simulink model "dec_fir_xblock"  (Simulink 7.4)
settings: Solver=ode45  StartTime=0.0  StopTime=10.0  RelTol=1e-3
libraries: xbsIndex_r4 x18, casper_library_misc x1
settings Model: Creator=chenhong  LastModifiedBy=chenhong

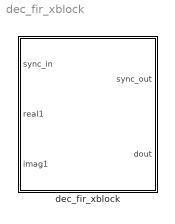
== system dec_fir_xblock ==
  dec_fir_xblock : Subsystem  mask{n_inputs=1, coeff=[0 0], n_bits=4, quantization=Truncate, add_latency=1, mult_latency=2, coeff_bit_width=25, coeff_bin_pt=24, adder_tree_hdl=on}
      mask prompts: n_inputs "Number of Parallel Streams"; coeff "Coefficients"; n_bits "Bit Width Out"; quantization "Quantization Behavior"; add_latency "Add Latency"; mult_latency "Mult Latency"; coeff_bit_width "Coefficient bit width"; coeff_bin_pt "Coefficient binary point"; adder_tree_hdl "Implement first stage of adder trees after multiplication as behavioural HDL"
      mask init:
      | config.source=str2func('dec_fir_init_xblock');
      | config.toplevel=gcb;
      | xBlock(config, ...
      |         {n_inputs,coeff,n_bits,quantization,add_latency,...
      |          mult_latency, coeff_bit_width,coeff_bin_pt,adder_tree_hdl})
      mask StyleString: edit,edit,edit,popup(Truncate|Round  (unbiased: +/- Inf)|Round  (unbiased: Even Values)),edit,edit,edit,edit,checkbox

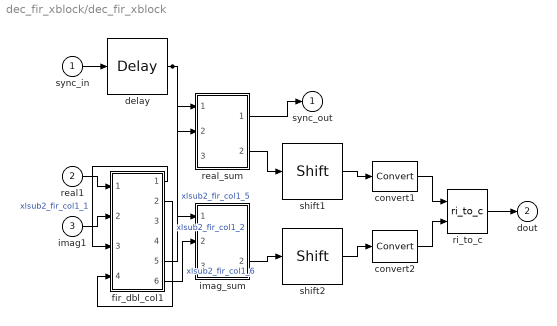
== system dec_fir_xblock/dec_fir_xblock ==
  sync_in : Inport
  real1 : Inport  Port=2
  imag1 : Inport  Port=3
  convert1 : xbsIndex_r4/Convert  arith_type="Signed  (2's comp)"  n_bits=4  bin_pt=3  quantization=Truncate  overflow=Wrap  latency=1  dbl_ovrd=off  pipeline=off  block_type=convert
      settings: block_version=11.4
  convert2 : xbsIndex_r4/Convert  arith_type="Signed  (2's comp)"  n_bits=4  bin_pt=3  quantization=Truncate  overflow=Wrap  latency=1  dbl_ovrd=off  pipeline=off  block_type=convert
      settings: block_version=11.4
  delay : xbsIndex_r4/Delay  en=off  latency=4  dbl_ovrd=off  reg_retiming=off  block_type=delay
      settings: block_version=11.4
  fir_dbl_col1 : Subsystem
  imag_sum : Subsystem
  real_sum : Subsystem
  ri_to_c : casper_library_misc/ri_to_c  SystemSampleTime=-1
  shift1 : xbsIndex_r4/Shift  shift_dir=Left  shift_bits=1  en=off  latency=0  precision=Full  arith_type="Signed  (2's comp)"  n_bits=16  bin_pt=14  quantization=Truncate  overflow=Wrap  dbl_ovrd=off  block_type=shift
  shift2 : xbsIndex_r4/Shift  shift_dir=Left  shift_bits=1  en=off  latency=0  precision=Full  arith_type="Signed  (2's comp)"  n_bits=16  bin_pt=14  quantization=Truncate  overflow=Wrap  dbl_ovrd=off  block_type=shift
  sync_out : Outport
  dout : Outport  Port=2
  wires:
  delay/1 -> real_sum/1(sync), imag_sum/1(sync)
  shift2/1 -> convert2/1
  imag_sum/2(dout) -> shift2/1
  shift1/1 -> convert1/1
  real_sum/2(dout) -> shift1/1
  ri_to_c/1 -> dout/1
  convert2/1 -> ri_to_c/2
  convert1/1 -> ri_to_c/1
  real_sum/1(sync_out) -> sync_out/1
  fir_dbl_col1/5(real_sum) -> real_sum/2(din_1)  "xlsub2_fir_col1_5"
  fir_dbl_col1/6(imag_sum) -> imag_sum/2(din_1)  "xlsub2_fir_col1_6"
  fir_dbl_col1/2(imag_out1) -> fir_dbl_col1/4(imag_back1)  "xlsub2_fir_col1_2"
  fir_dbl_col1/1(real_out1) -> fir_dbl_col1/3(real_back1)  "xlsub2_fir_col1_1"
  imag1/1 -> fir_dbl_col1/2(imag1)
  real1/1 -> fir_dbl_col1/1(real1)
  sync_in/1 -> delay/1

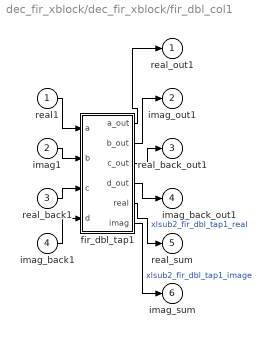
== system dec_fir_xblock/dec_fir_xblock/fir_dbl_col1 ==
  real1 : Inport
  imag1 : Inport  Port=2
  real_back1 : Inport  Port=3
  imag_back1 : Inport  Port=4
  fir_dbl_tap1 : Subsystem
  real_out1 : Outport
  imag_out1 : Outport  Port=2
  real_back_out1 : Outport  Port=3
  imag_back_out1 : Outport  Port=4
  real_sum : Outport  Port=5
  imag_sum : Outport  Port=6
  wires:
  fir_dbl_tap1/6(imag) -> imag_sum/1  "xlsub2_fir_dbl_tap1_image"
  fir_dbl_tap1/5(real) -> real_sum/1  "xlsub2_fir_dbl_tap1_real"
  fir_dbl_tap1/4(d_out) -> imag_back_out1/1
  fir_dbl_tap1/3(c_out) -> real_back_out1/1
  fir_dbl_tap1/2(b_out) -> imag_out1/1
  fir_dbl_tap1/1(a_out) -> real_out1/1
  imag_back1/1 -> fir_dbl_tap1/4(d)
  real_back1/1 -> fir_dbl_tap1/3(c)
  imag1/1 -> fir_dbl_tap1/2(b)
  real1/1 -> fir_dbl_tap1/1(a)

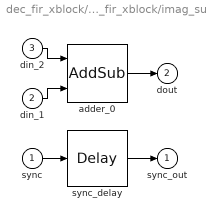
== system dec_fir_xblock/dec_fir_xblock/imag_sum ==
  sync : Inport
  din_1 : Inport  Port=2
  din_2 : Inport  Port=3
  adder_0 : xbsIndex_r4/AddSub  mode=Addition  use_carryin=off  use_carryout=off  en=off  latency=1  precision=Full  arith_type=Unsigned  n_bits=16  bin_pt=14  quantization=Truncate  overflow=Wrap  dbl_ovrd=off  use_behavioral_HDL=off  hw_selection=Fabric  pipelined=off  block_type=addsub
  sync_delay : xbsIndex_r4/Delay  en=off  latency=1  dbl_ovrd=off  reg_retiming=off  block_type=delay
      settings: block_version=11.4
  sync_out : Outport
  dout : Outport  Port=2
  wires:
  adder_0/1 -> dout/1
  din_1/1 -> adder_0/2
  din_2/1 -> adder_0/1
  sync_delay/1 -> sync_out/1
  sync/1 -> sync_delay/1

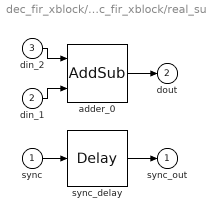
== system dec_fir_xblock/dec_fir_xblock/real_sum ==
  sync : Inport
  din_1 : Inport  Port=2
  din_2 : Inport  Port=3
  adder_0 : xbsIndex_r4/AddSub  mode=Addition  use_carryin=off  use_carryout=off  en=off  latency=1  precision=Full  arith_type=Unsigned  n_bits=16  bin_pt=14  quantization=Truncate  overflow=Wrap  dbl_ovrd=off  use_behavioral_HDL=off  hw_selection=Fabric  pipelined=off  block_type=addsub
  sync_delay : xbsIndex_r4/Delay  en=off  latency=1  dbl_ovrd=off  reg_retiming=off  block_type=delay
      settings: block_version=11.4
  sync_out : Outport
  dout : Outport  Port=2
  wires:
  adder_0/1 -> dout/1
  din_1/1 -> adder_0/2
  din_2/1 -> adder_0/1
  sync_delay/1 -> sync_out/1
  sync/1 -> sync_delay/1

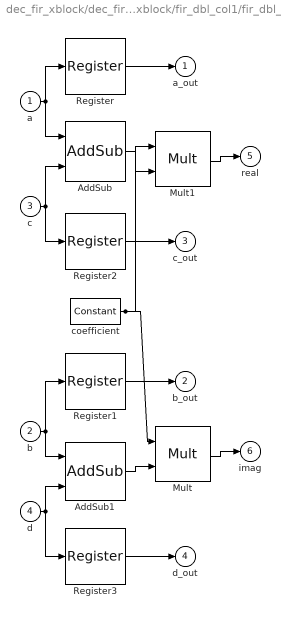
== system dec_fir_xblock/dec_fir_xblock/fir_dbl_col1/fir_dbl_tap1 ==
  a : Inport
  b : Inport  Port=2
  c : Inport  Port=3
  d : Inport  Port=4
  AddSub : xbsIndex_r4/AddSub  mode=Addition  use_carryin=off  use_carryout=off  en=off  latency=2  precision=Full  arith_type="Signed  (2's comp)"  n_bits=18  bin_pt=16  quantization=Truncate  overflow=Wrap  dbl_ovrd=off  use_behavioral_HDL=on  hw_selection=Fabric  pipelined=off  use_rpm=on  block_type=addsub
  AddSub1 : xbsIndex_r4/AddSub  mode=Addition  use_carryin=off  use_carryout=off  en=off  latency=2  precision=Full  arith_type="Signed  (2's comp)"  n_bits=18  bin_pt=16  quantization=Truncate  overflow=Wrap  dbl_ovrd=off  use_behavioral_HDL=on  hw_selection=Fabric  pipelined=off  use_rpm=on  block_type=addsub
  Mult : xbsIndex_r4/Mult  precision=Full  arith_type="Signed  (2's comp)"  n_bits=18  bin_pt=17  quantization=Truncate  overflow=Wrap  en=off  latency=1  dbl_ovrd=off  use_behavioral_HDL=on  opt=Speed  use_embedded=on  optimum_pipeline=off  pipeline=on  use_rpm=off  placement_style=Rectangular shape  block_type=mult
      settings: block_version=11.4
  Mult1 : xbsIndex_r4/Mult  precision=Full  arith_type="Signed  (2's comp)"  n_bits=18  bin_pt=17  quantization=Truncate  overflow=Wrap  en=off  latency=1  dbl_ovrd=off  use_behavioral_HDL=on  opt=Speed  use_embedded=on  optimum_pipeline=off  pipeline=on  use_rpm=off  placement_style=Rectangular shape  block_type=mult
      settings: block_version=11.4
  Register{,1..3} (4 alike) : xbsIndex_r4/Register  init=0  rst=off  en=off  dbl_ovrd=off  block_type=register
      settings: block_version=11.4
  coefficient : xbsIndex_r4/Constant  arith_type=Signed (2's comp)  const=0  n_bits=25  bin_pt=24  explicit_period=on  period=1  equ=P=C  opselect=C  inp2=PCIN>>17  opr=+  inp1=P  carry=CIN  dbl_ovrd=off  block_type=constant
      settings: block_version=11.4
  a_out : Outport
  b_out : Outport  Port=2
  c_out : Outport  Port=3
  d_out : Outport  Port=4
  real : Outport  Port=5
  imag : Outport  Port=6
  wires:
  a/1 -> Register/1, AddSub/1
  c/1 -> Register2/1, AddSub/2
  b/1 -> Register1/1, AddSub1/1
  d/1 -> Register3/1, AddSub1/2
  coefficient/1 -> Mult1/1, Mult/1
  Register3/1 -> d_out/1
  Register2/1 -> c_out/1
  Register1/1 -> b_out/1
  Register/1 -> a_out/1
  Mult1/1 -> real/1
  AddSub/1 -> Mult1/2
  Mult/1 -> imag/1
  AddSub1/1 -> Mult/2
